simulink model "logicGate"  (R2015a)
settings: Solver=ode1  StartTime=0.0  StopTime=10.0  FixedStep=1  RelTol=1e-3
settings Model: Creator=Osmaz  LastModifiedBy=Osmaz

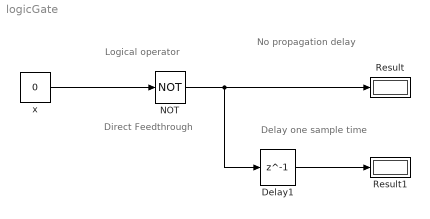
== system logicGate ==
  note: Direct Feedthrough
  note: Delay one sample time
  note: Logical operator
  note: No propagation delay
  Delay1 : Delay  DelayLength=1  InitialCondition=0  InputProcessing=Inherited
  NOT : Logic  Operator=NOT  IconShape=distinctive  AllPortsSameDT=off  OutDataTypeStr=boolean
  Result : Display
  Result1 : Display
  x : Constant  Value=0  OutMin=-8  OutMax=7  OutDataTypeStr=int8  SampleTime=1
  wires:
  NOT/1 -> Delay1/1, Result/1
  x/1 -> NOT/1
  Delay1/1 -> Result1/1
